simulink model "ValveHarness"  (R2023a)
settings: Solver=VariableStepAuto  StartTime=0.0  StopTime=10.0  RelTol=1e-3  AbsTol=1e-3
libraries: fl_lib x12, nesl_utility x6, SimscapeFluids_lib x3, simulink x1
CloseFcn:
  | try,close(h1_step5_ValveHarness),end
  | clear h1_step5_ValveHarness
  | try,close(h2_step5_ValveHarness),end
  | clear h2_step5_ValveHarness
  | try,close(h3_step5_ValveHarness),end
  | clear h3_step5_ValveHarness
  | try,close(h4_step5_ValveHarness),end
  | clear h4_step5_ValveHarness
  | 
  | 
  | clear simlog_step5_ValveHarness
  | clear logsout_step5_ValveHarness
settings Model: Creator=emcgarri  LastModifiedBy=esmithzb
settings SolverCC: AutoScaleAbsTol=off  AlgebraicLoopSolver=TrustRegion  MaxZcPerStep=1
settings DataIOCC: MaxDataPoints=10000  SignalLoggingName=logsout_ValveHarness
settings OptimizationCC: ReuseModelBlockBuffer=off
settings DebuggingCC: UnconnectedInputMsg=warning  UnconnectedOutputMsg=warning  UnconnectedLineMsg=warning  SymbolicDimsDataTypeCodeGenerationDiagnostic=none
settings ModelReferenceCC: EnableRefExpFcnMdlSchedulingChecks=on
settings SFSimCC: CustomCodeUndefinedFunction=UseInterfaceOnly
settings RTWCC: DLArmComputeVersion=19.05
settings SimscapeCC: SimscapeLogType=all  SimscapeLogSimulationStatistics=on  SimscapeLogName=simlog_ValveHarness  SimscapeLogDataHistory=10000

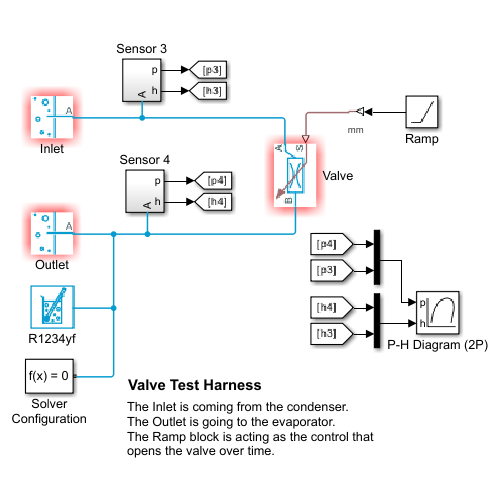
[thumbnail: Simulink's stored preview of the top-level diagram]
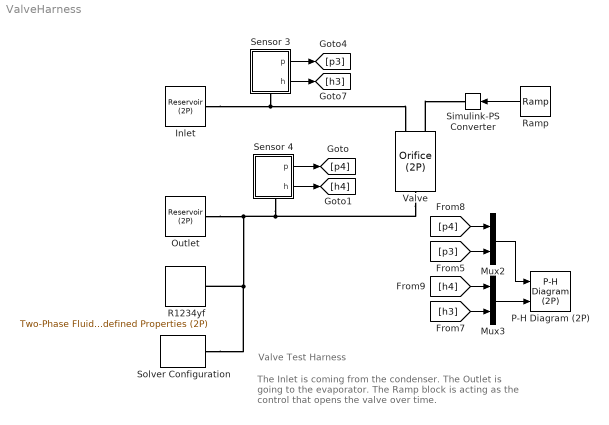
== system ValveHarness ==
  note: The Inlet is coming from the condenser.
      | The Outlet is going to the evaporator.
      | The Ramp block is acting as the control that
      | opens the valve over time.
  note: Valve Test Harness
  Inlet : fl_lib/Two-Phase Fluid/Elements/Reservoir (2P)  pressure_spec=foundation.enum.ReservoirPressureSpec2P.Specified  reservoir_pressure=p0_valve kPa  reservoir_condensing_temperature=373.15 K  reservoir_evaporating_temperature=373.15 K  energy_spec=foundation.enum.ReservoirEnergySpec2P.Enthalpy  reservoir_temperature=293.15 K  reservoir_quality=0.5  reservoir_void_fraction=0.5  reservoir_enthalpy=h0_valve kJ/kg  reservoir_internal_energy=1500 kJ/kg  reservoir_subcooling=5 deltaK  reservoir_superheating=5 deltaK  area_A=a_cond cm^2
  Mux2 : Mux  Inputs=2
  Mux3 : Mux  Inputs=2
  Outlet : fl_lib/Two-Phase Fluid/Elements/Reservoir (2P)  pressure_spec=foundation.enum.ReservoirPressureSpec2P.Specified  reservoir_pressure=p1_valve kPa  reservoir_condensing_temperature=373.15 K  reservoir_evaporating_temperature=373.15 K  energy_spec=foundation.enum.ReservoirEnergySpec2P.Enthalpy  reservoir_temperature=293.15 K  reservoir_quality=0.5  reservoir_void_fraction=0.5  reservoir_enthalpy=h1_valve kJ/kg  reservoir_internal_energy=1500 kJ/kg  reservoir_subcooling=5 deltaK  reservoir_superheating=5 deltaK  area_A=a_evap cm^2
  P-H Diagram (2P) : SimscapeFluids_lib/Two-Phase Fluid/Utilities/P-H Diagram (2P)
  R1234yf : SimscapeFluids_lib/Two-Phase Fluid/Utilities/Two-Phase Fluid Predefined Properties (2P)  fluid=fluids.two_phase_fluid.utilities.enum.Fluid.R1234yf  p_atm=0.101325 MPa  properties_range_check=simscape.enum.assert.action.error  q_rev=0.01 Pa
  Ramp : simulink/Sources/Ramp  slope=-5/10  start=0  InitialOutput=5
  Sensor 3 : Subsystem
      settings: PortSchema="{\"entries\":[{\"content\":{\"sides\":[{\"content\":{\"connectorIds\":[]},\"type\":\"ConnectorPlacement.EquallySpacedRectSide\",\"uuid\":\"41884682-286e-4d7b-b79e-2bb874be6d6c\"},{\"content\":{\"connectorIds\":[\"Out1\",\"Out2\"],\"side\":\"RIGHT\"},\"type\":\"ConnectorPlacement.EquallySpacedRectSide\",\"uuid\":\"e56675d9-2074-4825-bab9-53a77e88fae1\"},{\"content\":{\"connectorIds\":[],\"side\":\"TOP\"},\"type\":\"ConnectorPlacement.EquallySpacedRectSide\",\"uuid\":\"d9e20e39-37a5-4433-815e-653b161a9b7a\"},{\"content\":{\"connectorIds\":[\"RConn1\"],\"side\":\"BOTTOM\"},\"type\":\"ConnectorPlacement.EquallySpacedRectSide\",\"uuid\":\"0555c588-c570-4675-98ed-67bd7b6059f1\"}]},\"type\":\"ConnectorPlacement.EquallySpacedConnector\",\"uuid\":\"f059132f-c690-4b18-9213-6a7b84329d34\"}],\"packageUris\":[\"http://schema.mathworks.com/mf0/Connector/R2020b\"],\"version\":\"1.0\"}"
  Sensor 4 : Subsystem
      settings: PortSchema="{\"entries\":[{\"content\":{\"sides\":[{\"content\":{\"connectorIds\":[]},\"type\":\"ConnectorPlacement.EquallySpacedRectSide\",\"uuid\":\"a2386ea4-012f-4d06-9e16-de8034e56d49\"},{\"content\":{\"connectorIds\":[\"Out1\",\"Out2\"],\"side\":\"RIGHT\"},\"type\":\"ConnectorPlacement.EquallySpacedRectSide\",\"uuid\":\"4fc9eed4-9b91-4b18-836c-5d3d8d2a2391\"},{\"content\":{\"connectorIds\":[],\"side\":\"TOP\"},\"type\":\"ConnectorPlacement.EquallySpacedRectSide\",\"uuid\":\"63029c34-9cdb-4cf2-9461-f217553f00ec\"},{\"content\":{\"connectorIds\":[\"RConn1\"],\"side\":\"BOTTOM\"},\"type\":\"ConnectorPlacement.EquallySpacedRectSide\",\"uuid\":\"d2d8df23-35c6-4520-b0d8-5e88f3a56513\"}]},\"type\":\"ConnectorPlacement.EquallySpacedConnector\",\"uuid\":\"7866b668-ed43-4d72-8909-92d3adf450d4\"}],\"packageUris\":[\"http://schema.mathworks.com/mf0/Connector/R2020b\"],\"version\":\"1.0\"}"
  Simulink-PS Converter : nesl_utility/Simulink-PS Converter  PhysicalDomain=network_engine_domain  SubClassName=ps_input  LeftPortType=input  RightPortType=output  PseudoPeriodic=off  Frequencies=[]  NoiseDistribution=none  NoiseParameters=[]  Unit=mm  AffineConversion=off  FilteringAndDerivatives=provide  SimscapeFilterOrder=1  InputFilterTimeConstant=0.001  UdotUserProvided=0
  Solver Configuration : nesl_utility/Solver Configuration  PhysicalDomain=network_engine_domain  SubClassName=solver  LeftPortType=input  RightPortType=generic  Tones=[]  Harmonics=[]  SimulateNoise=off  Profile=off  UseLocalSampling=off  EnableSwitchedLinearOptims=on  FrequencyDomain=off  UseCCode=off  RelTol=0.001  AbsTol=1e-06  MinStep=1e-09  ToWorkspace=off  RevertToSquareIcSolve=off  NumHomotopyIterations=100  PhasorMode=off  PhasorModeNumHarmonics=1  ConsistencySolver=NEWTON_XTOL_AFTER_FTOL  IndexReductionMethod=DerivativeReplacement  DoDC=on  ResidualTolerance=1e-09  ConsistencyTolSource=GLOBAL  ConsistencyAbsTol=0.001  ConsistencyRelTol=0.001  ConsistencyTolFactor=0.001  UseLocalSolver=off  LocalSolverChoice=NE_BACKWARD_EULER_ADVANCER  ResolveIndetEquations=on  FunctionEvalNumThread=1  LocalSolverSampleTime=0.001  DoFixedCost=off  MaxNonlinIter=3  MaxModeIter=2  ComputeImpulses=off  ImpulseIterations=2  LinearAlgebra=auto  LinearAlgebraNumThread=0  EquationFormulation=NE_TIME_EF  DelaysMemoryBudget=1024  AutomaticFiltering=on  FilteringTimeConstant=0.001  PartitionStorageMethod=AS_NEEDED  PartitionMemoryBudget=1024  PartitionMethod=ROBUST
  Valve : SimscapeFluids_lib/Two-Phase Fluid/Valves & Orifices/Orifice (2P)  orifice_type=foundation.enum.constant_variable.variable  mdot_nominal_constant=0.1 kg/s  delta_p_nominal_constant=0.001 MPa  S_min=0 mm  del_S=valve_max_open mm  open_orientation=fluids.two_phase_fluid.valves_orifices.enum.OrificeOrientation.Positive  mdot_nominal_max=valve_nom_flow kg/s  delta_p_nominal_max=valve_nom_dp kPa  energy_spec=foundation.enum.energy_spec.enthalpy  p_inlet=p0_valve kPa  T_inlet=300 K  x_inlet=0.5  alpha_inlet=0.5  h_inlet=h0_valve kJ/kg  u_inlet=1500 kJ/kg  area=a_cond cm^2  mdot_leak_fraction=1e-6  smoothing_factor=0.01  B_lam=0.999  tau_x=0.1 s
      settings: InternalSimscapePortConfiguration="{\"Bottom\":[],\"Left\":[{\"id\":\"A\",\"label\":\"A\",\"type\":\"foundation.two_phase_fluid.two_phase_fluid\"},{\"id\":\"S\",\"label\":\"S\",\"type\":\"input\"}],\"Right\":[{\"id\":\"B\",\"label\":\"B\",\"type\":\"foundation.two_phase_fluid.two_phase_fluid\"}],\"Top\":[]}"
  wires:
  Sensor 3/2(h) -> [h3]
  Sensor 3/1(p) -> [p3]
  Sensor 4/1(p) -> [p4]
  Sensor 4/2(h) -> [h4]
  Mux3/1 -> P-H Diagram (2P)/2
  Mux2/1 -> P-H Diagram (2P)/1
  [h3] -> Mux3/2
  [p4] -> Mux2/1
  [h4] -> Mux3/1
  [p3] -> Mux2/2
  Ramp/1 -> Simulink-PS Converter/1
  connections:
  Valve/LConn2 -- Simulink-PS Converter/RConn1
  Inlet/LConn1 -- Sensor 3/RConn1 -- Valve/LConn1
  Valve/RConn1 -- Sensor 4/RConn1 -- Solver Configuration/RConn1 -- R1234yf/RConn1 -- Outlet/LConn1

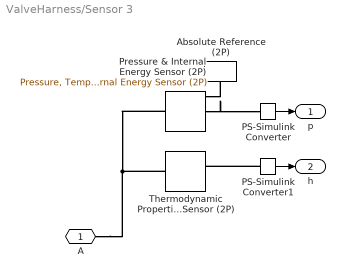
== system ValveHarness/Sensor 3 ==
  Absolute Reference (2P) : fl_lib/Two-Phase Fluid/Elements/Absolute Reference (2P)
  PS-Simulink Converter : nesl_utility/PS-Simulink Converter  PhysicalDomain=network_engine_domain  SubClassName=ps_output  LeftPortType=input  RightPortType=output  PseudoPeriodic=off  Frequencies=[]  VectorFormat=1-D array  Unit=MPa  AffineConversion=off
  PS-Simulink Converter1 : nesl_utility/PS-Simulink Converter  PhysicalDomain=network_engine_domain  SubClassName=ps_output  LeftPortType=input  RightPortType=output  PseudoPeriodic=off  Frequencies=[]  VectorFormat=1-D array  Unit=kJ/kg  AffineConversion=off
  Pressure & Internal Energy Sensor (2P) : fl_lib/Two-Phase Fluid/Sensors/Pressure, Temperature & Internal Energy Sensor (2P)  reference=foundation.enum.MeasurementReference.difference  pressure=true  pressure_spec=foundation.enum.PressureMeasementSpec.Absolute  temperature=false  internal_energy=true
      settings: InternalSimscapePortConfiguration="{\"Bottom\":[{\"id\":\"U\",\"label\":\"U\",\"type\":\"output\"}],\"Left\":[{\"id\":\"A\",\"label\":\"A\",\"type\":\"foundation.two_phase_fluid.two_phase_fluid\"}],\"Right\":[{\"id\":\"B\",\"label\":\"B\",\"type\":\"foundation.two_phase_fluid.two_phase_fluid\"},{\"id\":\"P\",\"label\":\"P\",\"type\":\"output\"}],\"Top\":[]}"
  Thermodynamic Properties Sensor (2P) : fl_lib/Two-Phase Fluid/Sensors/Thermodynamic Properties Sensor (2P)  temperature=true  enthalpy=true  density=false  specific_volume=true  entropy=true
      settings: InternalSimscapePortConfiguration="{\"Bottom\":[{\"id\":\"V\",\"label\":\"v\",\"type\":\"output\"},{\"id\":\"S\",\"label\":\"s\",\"type\":\"output\"}],\"Left\":[{\"id\":\"A\",\"label\":\"A\",\"type\":\"foundation.two_phase_fluid.two_phase_fluid\"}],\"Right\":[{\"id\":\"T\",\"label\":\"T\",\"type\":\"output\"},{\"id\":\"H\",\"label\":\"h\",\"type\":\"output\"}],\"Top\":[]}"
  A : PMIOPort  Side=Right
  p : Outport
  h : Outport  Port=2
  wires:
  PS-Simulink Converter/1 -> p/1
  PS-Simulink Converter1/1 -> h/1
  connections:
  Thermodynamic Properties Sensor (2P)/LConn1 -- Pressure & Internal Energy Sensor (2P)/LConn1 -- A/RConn1
  Pressure & Internal Energy Sensor (2P)/RConn2 -- PS-Simulink Converter/LConn1
  Pressure & Internal Energy Sensor (2P)/RConn1 -- Absolute Reference (2P)/LConn1
  PS-Simulink Converter1/LConn1 -- Thermodynamic Properties Sensor (2P)/RConn2

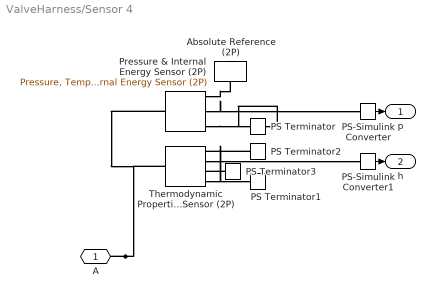
== system ValveHarness/Sensor 4 ==
  Absolute Reference (2P) : fl_lib/Two-Phase Fluid/Elements/Absolute Reference (2P)
  PS Terminator{,1..3} (4 alike) : fl_lib/Physical Signals/Sinks/PS Terminator
  PS-Simulink Converter : nesl_utility/PS-Simulink Converter  PhysicalDomain=network_engine_domain  SubClassName=ps_output  LeftPortType=input  RightPortType=output  PseudoPeriodic=off  Frequencies=[]  VectorFormat=1-D array  Unit=MPa  AffineConversion=off
  PS-Simulink Converter1 : nesl_utility/PS-Simulink Converter  PhysicalDomain=network_engine_domain  SubClassName=ps_output  LeftPortType=input  RightPortType=output  PseudoPeriodic=off  Frequencies=[]  VectorFormat=1-D array  Unit=kJ/kg  AffineConversion=off
  Pressure & Internal Energy Sensor (2P) : fl_lib/Two-Phase Fluid/Sensors/Pressure, Temperature & Internal Energy Sensor (2P)  reference=foundation.enum.MeasurementReference.difference  pressure=true  pressure_spec=foundation.enum.PressureMeasementSpec.Absolute  temperature=false  internal_energy=true
      settings: InternalSimscapePortConfiguration="{\"Bottom\":[{\"id\":\"U\",\"label\":\"U\",\"type\":\"output\"}],\"Left\":[{\"id\":\"A\",\"label\":\"A\",\"type\":\"foundation.two_phase_fluid.two_phase_fluid\"}],\"Right\":[{\"id\":\"B\",\"label\":\"B\",\"type\":\"foundation.two_phase_fluid.two_phase_fluid\"},{\"id\":\"P\",\"label\":\"P\",\"type\":\"output\"}],\"Top\":[]}"
  Thermodynamic Properties Sensor (2P) : fl_lib/Two-Phase Fluid/Sensors/Thermodynamic Properties Sensor (2P)  temperature=true  enthalpy=true  density=false  specific_volume=true  entropy=true
      settings: InternalSimscapePortConfiguration="{\"Bottom\":[{\"id\":\"V\",\"label\":\"v\",\"type\":\"output\"},{\"id\":\"S\",\"label\":\"s\",\"type\":\"output\"}],\"Left\":[{\"id\":\"A\",\"label\":\"A\",\"type\":\"foundation.two_phase_fluid.two_phase_fluid\"}],\"Right\":[{\"id\":\"T\",\"label\":\"T\",\"type\":\"output\"},{\"id\":\"H\",\"label\":\"h\",\"type\":\"output\"}],\"Top\":[]}"
  A : PMIOPort  Side=Right
  p : Outport
  h : Outport  Port=2
  wires:
  PS-Simulink Converter/1 -> p/1
  PS-Simulink Converter1/1 -> h/1
  connections:
  Thermodynamic Properties Sensor (2P)/RConn4 -- PS Terminator1/LConn1
  Pressure & Internal Energy Sensor (2P)/RConn1 -- Absolute Reference (2P)/LConn1
  A/RConn1 -- Pressure & Internal Energy Sensor (2P)/LConn1 -- Thermodynamic Properties Sensor (2P)/LConn1
  Pressure & Internal Energy Sensor (2P)/RConn3 -- PS Terminator/LConn1
  PS Terminator3/LConn1 -- Thermodynamic Properties Sensor (2P)/RConn3
  Pressure & Internal Energy Sensor (2P)/RConn2 -- PS-Simulink Converter/LConn1
  PS Terminator2/LConn1 -- Thermodynamic Properties Sensor (2P)/RConn1
  Thermodynamic Properties Sensor (2P)/RConn2 -- PS-Simulink Converter1/LConn1
